simulink model "lab1_only_PD_2"  (Simulink 7.2)
settings: Solver=ode45  StartTime=0.0  StopTime=10  RelTol=1e-3
values from neighbouring files (symbols this model uses):
  g = 9.81    [Variables_001.m]
  l = 1    [Variables_001.m]
  M = 10    [Variables_001.m]
  m = 1    [Variables_001.m]
  q0 = 0.1    [Variables_001.m]
settings Model: Creator=Student  LastModifiedBy=Student
settings SolverCC: ZcThreshold=0.01  MaxConsecutiveZCs=100  ZeroCrossAlgorithm=Adaptive
settings DataIOCC: SignalLoggingName=SDO_logsout
settings OptimizationCC: ExpressionDepthLimit=128
settings DebuggingCC: AlgebraicLoopMsg=error  UnderspecifiedInitializationDetection=Simplified  MergeDetectMultiDrivingBlocksExec=error  SolverPrmCheckMsg=none  FcnCallInpInsideContextMsg=Enable All  StateNameClashWarn=none  StrictBusMsg=ErrorLevel1
settings HardwareCC: ProdBitPerLong=64  ProdIntDivRoundTo=Zero  ProdEndianess=LittleEndian  ProdWordSize=64  ProdHWDeviceType=Intel->x86-64
settings RTWCC: Description=Create Visual C/C++ Solution File for Simulink Coder  GenerateReport=on  RetainRTWFile=on  LaunchReport=on
settings CodeAppCC: ForceParamTrailComments=on  CustomSymbolStrType=$N$R$M_T
settings GRTTargetCC: TargetFunctionLibrary=C99 (ISO)

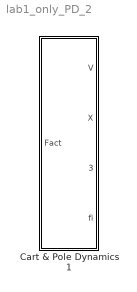
== system lab1_only_PD_2 ==
  Cart & Pole Dynamics 1 : Subsystem

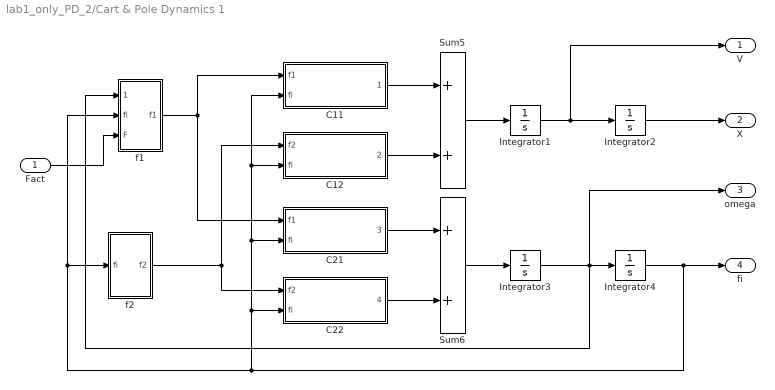
== system lab1_only_PD_2/Cart & Pole Dynamics 1 ==
  Fact : Inport
  C11 : Subsystem
  C12 : Subsystem
  C21 : Subsystem
  C22 : Subsystem
  Integrator1 : Integrator
  Integrator2 : Integrator
  Integrator3 : Integrator
  Integrator4 : Integrator  InitialCondition=q0
  Sum5 : Sum
  Sum6 : Sum
  f1 : Subsystem
  f2 : Subsystem
  V : Outport
  X : Outport  Port=2
  omega : Outport  Port=3
  fi : Outport  Port=4
  wires:
  Sum5/1 -> Integrator1/1
  C12/1(2) -> Sum5/2
  C22/1(4) -> Sum6/2
  C21/1(3) -> Sum6/1
  Sum6/1 -> Integrator3/1
  C11/1(1) -> Sum5/1
  Integrator2/1 -> X/1
  Integrator3/1 -> f1/1(omega), omega/1, Integrator4/1
  Integrator1/1 -> V/1, Integrator2/1
  Fact/1 -> f1/3(F)
  f1/1(f1) -> C21/1(f1), C11/1(f1)
  f2/1(f2) -> C22/1(f2), C12/1(f2)
  Integrator4/1 -> f2/1(fi), f1/2(fi), C22/2(fi), C21/2(fi), C12/2(fi), C11/2(fi), fi/1

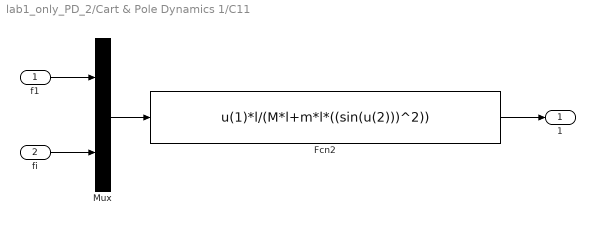
== system lab1_only_PD_2/Cart & Pole Dynamics 1/C11 ==
  f1 : Inport
  fi : Inport  Port=2
  Fcn2 : Fcn  Expr=u(1)*l/(M*l+m*l*((sin(u(2)))^2))
  Mux : Mux  Inputs=2
  1 : Outport
  wires:
  f1/1 -> Mux/1
  Mux/1 -> Fcn2/1
  fi/1 -> Mux/2
  Fcn2/1 -> 1/1

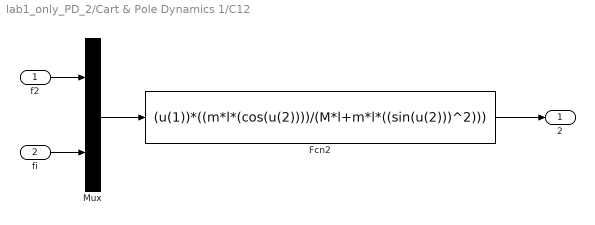
== system lab1_only_PD_2/Cart & Pole Dynamics 1/C12 ==
  f2 : Inport
  fi : Inport  Port=2
  Fcn2 : Fcn  Expr=(u(1))*((m*l*(cos(u(2))))/(M*l+m*l*((sin(u(2)))^2)))
  Mux : Mux  Inputs=2
  2 : Outport
  wires:
  f2/1 -> Mux/1
  Mux/1 -> Fcn2/1
  Fcn2/1 -> 2/1
  fi/1 -> Mux/2

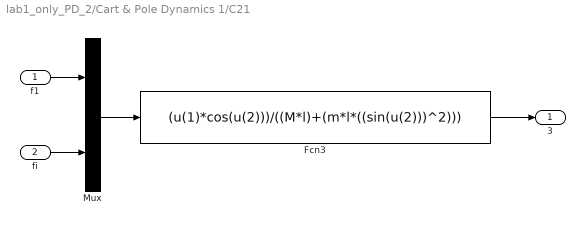
== system lab1_only_PD_2/Cart & Pole Dynamics 1/C21 ==
  f1 : Inport
  fi : Inport  Port=2
  Fcn3 : Fcn  Expr=(u(1)*cos(u(2)))/((M*l)+(m*l*((sin(u(2)))^2)))
  Mux : Mux  Inputs=2
  3 : Outport
  wires:
  f1/1 -> Mux/1
  Mux/1 -> Fcn3/1
  Fcn3/1 -> 3/1
  fi/1 -> Mux/2

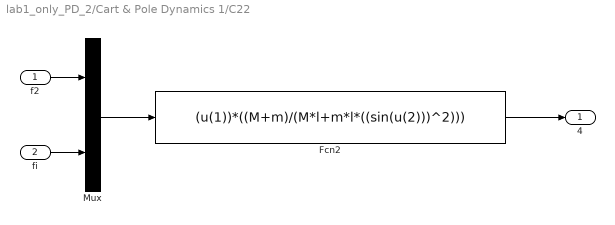
== system lab1_only_PD_2/Cart & Pole Dynamics 1/C22 ==
  f2 : Inport
  fi : Inport  Port=2
  Fcn2 : Fcn  Expr=(u(1))*((M+m)/(M*l+m*l*((sin(u(2)))^2)))
  Mux : Mux  Inputs=2
  4 : Outport
  wires:
  f2/1 -> Mux/1
  Mux/1 -> Fcn2/1
  Fcn2/1 -> 4/1
  fi/1 -> Mux/2

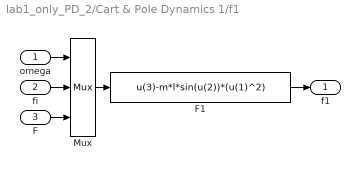
== system lab1_only_PD_2/Cart & Pole Dynamics 1/f1 ==
  omega : Inport
  fi : Inport  Port=2
  F : Inport  Port=3
  F1 : Fcn  Expr=u(3)-m*l*sin(u(2))*(u(1)^2)
  Mux : Mux  Inputs=3
  f1 : Outport
  wires:
  F1/1 -> f1/1
  Mux/1 -> F1/1
  fi/1 -> Mux/2
  F/1 -> Mux/3
  omega/1 -> Mux/1

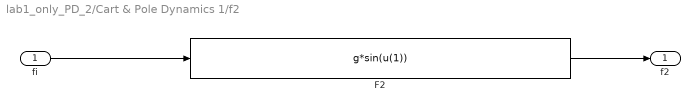
== system lab1_only_PD_2/Cart & Pole Dynamics 1/f2 ==
  fi : Inport
  F2 : Fcn  Expr=g*sin(u(1))
  f2 : Outport
  wires:
  fi/1 -> F2/1
  F2/1 -> f2/1
